simulink model "adrcsim"  (R2018a)
settings: Solver=ode4  StartTime=0.0  StopTime=3  FixedStep=1/30e3  RelTol=1e-3  EnableMultiTasking=on
undefined symbols (not defined in the file): DiscIntNeverNeededParam, MotorParams, Obs_K1, Obs_K2, Obs_K3
libraries: ctrl_lib x2
settings Model: PauseTimes=0.1  Creator=uids8840  LastModifiedBy=elrobotista
settings SolverCC: AlgebraicLoopSolver=LineSearch
settings DataIOCC: LimitDataPoints=on  SaveFormat=Array  SaveOutput=off  DSMLogging=off  SaveTime=off
settings OptimizationCC: DefaultParameterBehavior=Inlined  UseFloatMulNetSlope=on  DefaultUnderspecifiedDataType=single  InlineInvariantSignals=on  PassReuseOutputArgsAs=Individual arguments  ZeroExternalMemoryAtStartup=off  ZeroInternalMemoryAtStartup=off  NoFixptDivByZeroProtection=on  EfficientFloat2IntCast=on  LifeSpan=1
settings DebuggingCC: SolverPrmCheckMsg=warning  MultiTaskRateTransMsg=warning  ParameterTunabilityLossMsg=error  SFUnexpectedBacktrackingDiag=warning  SFNoUnconditionalDefaultTransitionDiag=warning  SFExecutionAtInitializationDiag=none
settings HardwareCC: ProdBitPerPointer=32  ProdBitPerSizeT=32  ProdBitPerPtrDiffT=32  ProdLargestAtomicInteger=Long  ProdLargestAtomicFloat=Double  ProdWordSize=32  ProdHWDeviceType=ARM Compatible->ARM Cortex
settings ModelReferenceCC: UpdateModelReferenceTargets=IfOutOfDate  EnableRefExpFcnMdlSchedulingChecks=off  ModelReferenceNumInstancesAllowed=Single  PropagateSignalLabelsOutOfModel=off
settings SFSimCC: SFSimEcho=off  SimCtrlC=off  SimIntegrity=off  MATLABDynamicMemAlloc=off
settings RTWCC: SystemTargetFile=ert.tlc  TemplateMakefile=ert_default_tmf  GenerateReport=on  IncludeHyperlinkInReport=on  LaunchReport=on  GenerateTraceInfo=on  GenerateTraceReport=on  GenerateTraceReportSl=on  GenerateTraceReportSf=on  GenerateTraceReportEml=on  GenerateCodeMetricsReport=on
settings CodeAppCC: ForceParamTrailComments=on  IgnoreCustomStorageClasses=off  OperatorAnnotations=on  SimulinkDataObjDesc=on  SFDataObjDesc=on  CustomSymbolStrGlobalVar=rt$N$M  CustomSymbolStrType=$N$M  CustomSymbolStrFcn=$N$M$F  CustomSymbolStrMacro=$N$M  InsertBlockDesc=on  StateflowObjectComments=on
settings ERTTargetCC: GenerateSampleERTMain=on  IncludeMdlTerminateFcn=off  CombineSignalStateStructs=on  SupportComplex=off  InlinedParameterPlacement=NonHierarchical  ERTCustomFileTemplate=example_file_process.tlc
settings ConfigComp: CovMetricSettings=dw  CovHtmlReporting=on  CovSaveCumulativeToWorkspaceVar=on  CovSaveSingleToWorkspaceVar=on  CovExternalEMLEnable=off

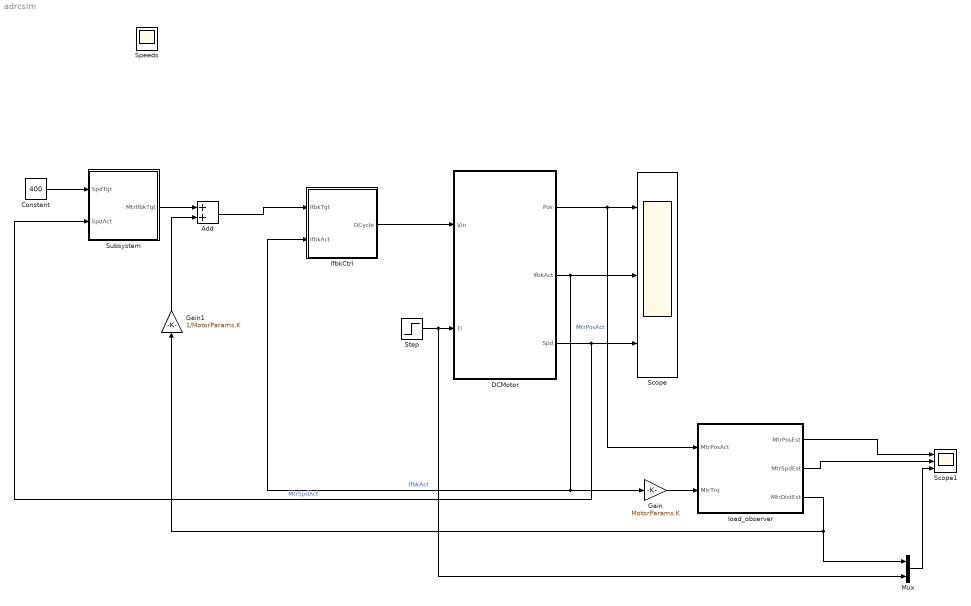
== system adrcsim ==
  Add : Sum
  Constant : Constant  Value=400
  DCMotor : Subsystem
  Gain : Gain  Gain=MotorParams.K
  Gain1 : Gain  Gain=1/MotorParams.K
  IfbkCtrl : Subsystem  TreatAsAtomicUnit=on  SystemSampleTime=1/30e3
  Mux : Mux  Inputs=2
  Scope : Scope  NumInputPorts=3
  Scope1 : Scope  NumInputPorts=3
  Step : Step  After=4e-3  SampleTime=0
  Subsystem : Subsystem  TreatAsAtomicUnit=on  SystemSampleTime=1e-3
  load_observer : Subsystem  TreatAsAtomicUnit=on  SystemSampleTime=1/30e3
  Speeds : Scope
  wires:
  DCMotor/3(Spd) -> Subsystem/2(SpdAct), Scope/3  "MtrSpdAct"
  DCMotor/2(IfbkAct) -> IfbkCtrl/2(IfbkAct), Gain/1, Scope/2  "IfbkAct"
  DCMotor/1(Pos) -> load_observer/1(MtrPosAct), Scope/1  "MtrPosAct"
  IfbkCtrl/1(DCycle) -> DCMotor/1(Vin)
  Step/1 -> Mux/2, DCMotor/2(Tl)
  Constant/1 -> Subsystem/1(SpdTgt)
  load_observer/1(MtrPosEst) -> Scope1/1
  load_observer/2(MtrSpdEst) -> Scope1/2
  load_observer/3(MtrDistEst) -> Mux/1, Gain1/1
  Gain/1 -> load_observer/2(MtrTrq)
  Subsystem/1(MtrIfbkTgt) -> Add/1
  Add/1 -> IfbkCtrl/1(IfbkTgt)
  Gain1/1 -> Add/2
  Mux/1 -> Scope1/3

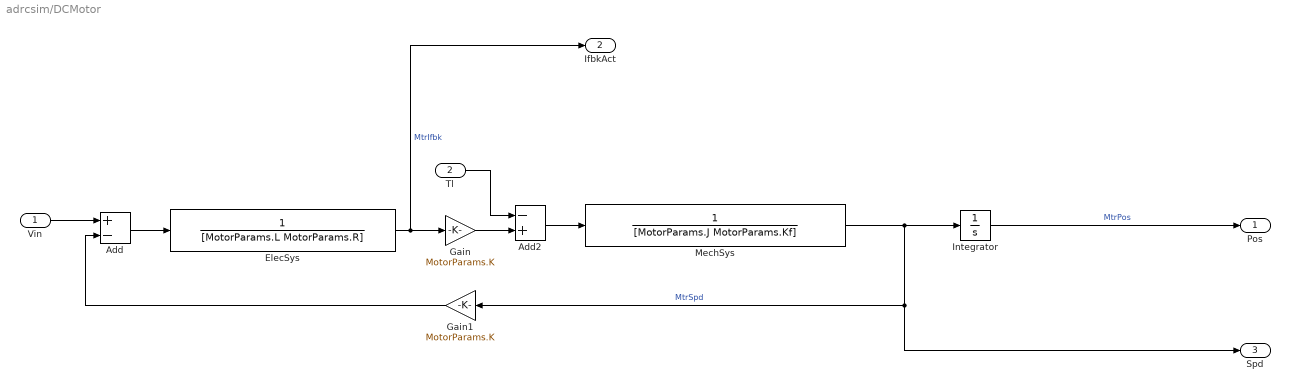
== system adrcsim/DCMotor ==
  Vin : Inport
  Tl : Inport  Port=2
  Add : Sum  Inputs=+-
  Add2 : Sum  Inputs=-+
  ElecSys : TransferFcn  Denominator=[MotorParams.L MotorParams.R]
  Gain : Gain  Gain=MotorParams.K
  Gain1 : Gain  Gain=MotorParams.K
  Integrator : Integrator
  MechSys : TransferFcn  Denominator=[MotorParams.J MotorParams.Kf]
  Pos : Outport
  IfbkAct : Outport  Port=2
  Spd : Outport  Port=3
  wires:
  ElecSys/1 -> IfbkAct/1, Gain/1  "MtrIfbk"
  MechSys/1 -> Gain1/1, Spd/1, Integrator/1  "MtrSpd"
  Add2/1 -> MechSys/1
  Tl/1 -> Add2/1
  Integrator/1 -> Pos/1  "MtrPos"
  Add/1 -> ElecSys/1
  Vin/1 -> Add/1
  Gain/1 -> Add2/2
  Gain1/1 -> Add/2

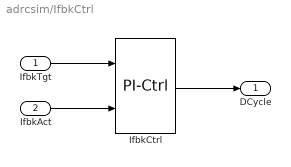
== system adrcsim/IfbkCtrl ==
  IfbkTgt : Inport
  IfbkAct : Inport  Port=2
  IfbkCtrl : ctrl_lib/PI-Ctrl  ts=TsFast  PI_Kp=IfbkCtrl_Kp  PI_Ki=IfbkCtrl_Ki  max_lim=12  min_lim=-12.
  DCycle : Outport
  wires:
  IfbkTgt/1 -> IfbkCtrl/1
  IfbkAct/1 -> IfbkCtrl/2
  IfbkCtrl/1 -> DCycle/1

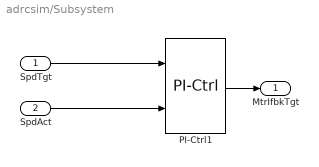
== system adrcsim/Subsystem ==
  SpdTgt : Inport
  SpdAct : Inport  Port=2
  PI-Ctrl1 : ctrl_lib/PI-Ctrl  ts=TsMain  PI_Kp=SpdCtrl_Kp  PI_Ki=SpdCtrl_Ki  max_lim=1.  min_lim=-1.
  MtrIfbkTgt : Outport
  wires:
  PI-Ctrl1/1 -> MtrIfbkTgt/1
  SpdAct/1 -> PI-Ctrl1/2
  SpdTgt/1 -> PI-Ctrl1/1

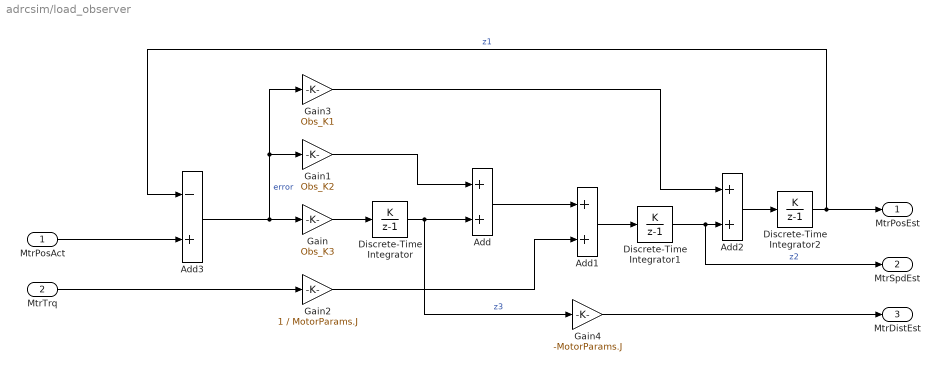
== system adrcsim/load_observer ==
  MtrPosAct : Inport
  MtrTrq : Inport  Port=2
  Add : Sum
  Add1 : Sum
  Add2 : Sum
  Add3 : Sum  Inputs=-+
  Discrete-Time Integrator : DiscreteIntegrator  IntegratorMethod=Accumulation: Forward Euler  gainval=1/30e3  SampleTime=-1  ICPrevOutput=DiscIntNeverNeededParam  ICPrevScaledInput=DiscIntNeverNeededParam
  Discrete-Time Integrator1 : DiscreteIntegrator  IntegratorMethod=Accumulation: Forward Euler  gainval=1/30e3  SampleTime=-1  ICPrevOutput=DiscIntNeverNeededParam  ICPrevScaledInput=DiscIntNeverNeededParam
  Discrete-Time Integrator2 : DiscreteIntegrator  IntegratorMethod=Accumulation: Forward Euler  gainval=1/30e3  SampleTime=-1  ICPrevOutput=DiscIntNeverNeededParam  ICPrevScaledInput=DiscIntNeverNeededParam
  Gain : Gain  Gain=Obs_K3
      settings: AttributesFormatString=%<Gain>
  Gain1 : Gain  Gain=Obs_K2
      settings: AttributesFormatString=%<Gain>
  Gain2 : Gain  Gain=1 / MotorParams.J
      settings: AttributesFormatString=%<Gain>
  Gain3 : Gain  Gain=Obs_K1
      settings: AttributesFormatString=%<Gain>
  Gain4 : Gain  Gain=-MotorParams.J
      settings: AttributesFormatString=%<Gain>
  MtrPosEst : Outport
  MtrSpdEst : Outport  Port=2
  MtrDistEst : Outport  Port=3
  wires:
  Gain4/1 -> MtrDistEst/1
  MtrTrq/1 -> Gain2/1
  Add3/1 -> Gain/1, Gain1/1, Gain3/1  "error"
  Gain2/1 -> Add1/2
  Add1/1 -> Discrete-Time Integrator1/1
  MtrPosAct/1 -> Add3/2
  Add2/1 -> Discrete-Time Integrator2/1
  Discrete-Time Integrator2/1 -> Add3/1, MtrPosEst/1  "z1"
  Gain/1 -> Discrete-Time Integrator/1
  Discrete-Time Integrator1/1 -> Add2/2, MtrSpdEst/1  "z2"
  Gain1/1 -> Add/1
  Discrete-Time Integrator/1 -> Add/2, Gain4/1  "z3"
  Add/1 -> Add1/1
  Gain3/1 -> Add2/1
